simulink model "SwitchingDecisionMechanism_v02"  (R2021a)
settings: Solver=FixedStepAuto  StartTime=0.0  StopTime=inf  RelTol=1e-3
model workspace (MAT data in the model file):
  SL_ROS_VariableLengthArrays_MaxSizes.CommonInfo.ArrayTruncateAction = 'EmitWarning'
  SL_ROS_VariableLengthArrays_MaxSizes.MsgTypeMap = containers.Map
  SL_ROS_VariableLengthArrays_MaxSizes.MsgTypeMap.serialization.keys = {'sensor_msgs/LaserScan'}
  SL_ROS_VariableLengthArrays_MaxSizes.MsgTypeMap.serialization.values{1}(1).PropertyName = 'Intensities'
  SL_ROS_VariableLengthArrays_MaxSizes.MsgTypeMap.serialization.values{1}(1).DataType = 'single'
  SL_ROS_VariableLengthArrays_MaxSizes.MsgTypeMap.serialization.values{1}(1).MaxLength = 1084
  SL_ROS_VariableLengthArrays_MaxSizes.MsgTypeMap.serialization.values{1}(2).PropertyName = 'Ranges'
  SL_ROS_VariableLengthArrays_MaxSizes.MsgTypeMap.serialization.values{1}(2).DataType = 'single'
  SL_ROS_VariableLengthArrays_MaxSizes.MsgTypeMap.serialization.values{1}(2).MaxLength = 1084
  SL_ROS_VariableLengthArrays_MaxSizes.MsgTypeMap.serialization.uniformity = 0
  SL_ROS_VariableLengthArrays_MaxSizes.MsgTypeMap.serialization.keyType = 'char'
  SL_ROS_VariableLengthArrays_MaxSizes.MsgTypeMap.serialization.valueType = 'any'
libraries: robotlib x3
settings Model: Creator=roboticlab01  LastModifiedBy=roboticlab02
settings SolverCC: AlgebraicLoopSolver=TrustRegion
settings OptimizationCC: EnhancedBackFolding=on  PassReuseOutputArgsAs=Individual arguments  MaxStackSize=64  OptimizeBlockOrder=speed  DifferentSizesBufferReuse=on  OptimizationCustomize=off  EfficientTunableParamExpr=on
settings DebuggingCC: ParameterTunabilityLossMsg=error  SFMachineParentedDataDiag=warning
settings HardwareCC: ProdBitPerPointer=32  ProdBitPerSizeT=32  ProdBitPerPtrDiffT=32  ProdLargestAtomicFloat=None  ProdIntDivRoundTo=Undefined  ProdEndianess=Unspecified  ProdWordSize=32  ProdHWDeviceType=Generic->Unspecified (assume 32-bit Generic)
settings SFSimCC: MATLABDynamicMemAlloc=off  CustomCodeUndefinedFunction=UseInterfaceOnly  SimTargetLang=C++
settings RTWCC: SystemTargetFile=ert.tlc  HardwareBoard=Robot Operating System (ROS)  TLCOptions="-aInlineSetEventsForThisBaseRateFcn=TLC_FALSE -aSuppressMultiTaskScheduler=TLC_FALSE  -aRateBasedStepFcn=0"  TemplateMakefile=ert_default_tmf  GenerateReport=on  Toolchain=Catkin  IncludeHyperlinkInReport=on  LaunchReport=on  TargetLang=C++  GenerateTraceInfo=on  GenerateTraceReport=on  GenerateTraceReportSl=on  GenerateTraceReportSf=on  GenerateTraceReportEml=on
settings CodeAppCC: ForceParamTrailComments=on  IgnoreCustomStorageClasses=off  OperatorAnnotations=on  SimulinkDataObjDesc=on  SFDataObjDesc=on  InsertBlockDesc=on
settings ERTTargetCC: SupportVariableSizeSignals=on

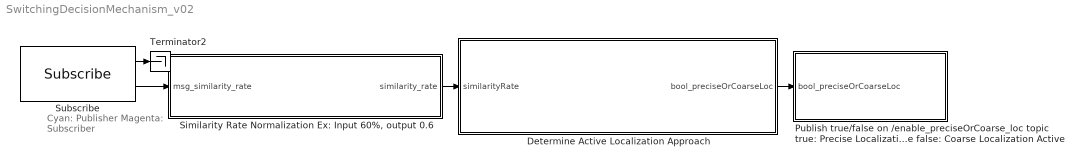
== system SwitchingDecisionMechanism_v02 ==
  note: Cyan: Publisher
      | Magenta: Subscriber
  Determine Active Localization Approach : Subsystem
  Publish true/false on /enable_preciseOrCoarse_loc topic true: Precise Localization Active false: Coarse Localization Active : Subsystem
  "Similarity Rate Normalization Ex: Input 60%, output 0.6" : Subsystem
  Subscribe : robotlib/Subscribe  topicSource=Specify your own  topic=/similarity_rate_corr  messageType=std_msgs/Int16  SampleTime=-1  legacyBusStruct=off  messageQueueLength=1
  Terminator2 : Terminator
  wires:
  Subscribe/1 -> Terminator2/1
  Subscribe/2 -> "Similarity Rate Normalization Ex: Input 60%, output 0.6"/1(msg_similarity_rate)
  "Similarity Rate Normalization Ex: Input 60%, output 0.6"/1(similarity_rate) -> Determine Active Localization Approach/1(similarityRate)
  Determine Active Localization Approach/1(bool_preciseOrCoarseLoc) -> Publish true/false on /enable_preciseOrCoarse_loc topic true: Precise Localization Active false: Coarse Localization Active/1(bool_preciseOrCoarseLoc)

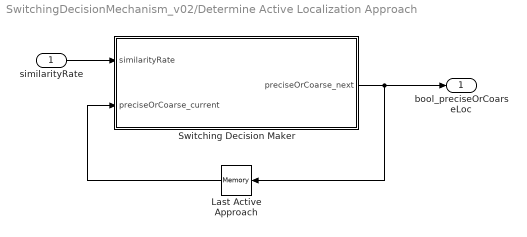
== system SwitchingDecisionMechanism_v02/Determine Active Localization Approach ==
  similarityRate : Inport
  Last Active Approach : Memory  InitialCondition=false(1)
  Switching Decision Maker : MATLAB Function  TreatAsAtomicUnit=on
  bool_preciseOrCoarseLoc : Outport
  wires:
  Switching Decision Maker/1(preciseOrCoarse_next) -> bool_preciseOrCoarseLoc/1, Last Active Approach/1
  similarityRate/1 -> Switching Decision Maker/1(similarityRate)
  Last Active Approach/1 -> Switching Decision Maker/2(preciseOrCoarse_current)

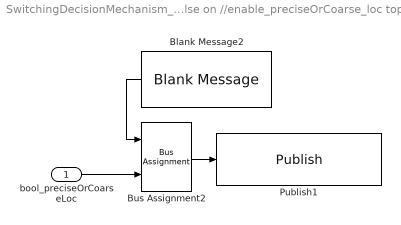
== system SwitchingDecisionMechanism_v02/Publish true//false on //enable_preciseOrCoarse_loc topic true: Precise Localization Active false: Coarse Localization Active ==
  bool_preciseOrCoarseLoc : Inport
  Blank Message2 : robotlib/Blank Message  messageClass=Message  entityType=std_msgs/Bool  messageType=std_msgs/Bool  SampleTime=inf  legacyBusStruct=off
      settings: SourceProductBaseCode=RO
  Bus Assignment2 : BusAssignment  AssignedSignals=Data
  Publish1 : robotlib/Publish  topicSource=Specify your own  topic=/enable_preciseOrCoarse_loc  messageType=std_msgs/Bool  legacyBusStruct=off  messageQueueLength=1
      settings: SourceProductBaseCode=RO
  wires:
  Bus Assignment2/1 -> Publish1/1
  bool_preciseOrCoarseLoc/1 -> Bus Assignment2/2
  Blank Message2/1 -> Bus Assignment2/1

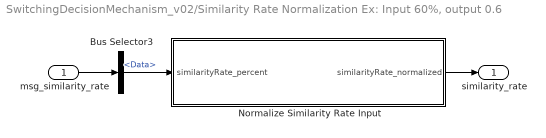
== system SwitchingDecisionMechanism_v02/Similarity Rate Normalization Ex: Input 60%, output 0.6 ==
  msg_similarity_rate : Inport
  Bus Selector3 : BusSelector  OutputSignals=Data
  Normalize Similarity Rate Input : MATLAB Function  TreatAsAtomicUnit=on
  similarity_rate : Outport
  wires:
  Bus Selector3/1 -> Normalize Similarity Rate Input/1(similarityRate_percent)  "<Data>"
  msg_similarity_rate/1 -> Bus Selector3/1
  Normalize Similarity Rate Input/1(similarityRate_normalized) -> similarity_rate/1

== matlab function SwitchingDecisionMechanism_v02/Determine Active Localization Approach/Switching Decision Maker ==
  data: similarityRate input; preciseOrCoarse_current input; preciseOrCoarse_next output
function preciseOrCoarse_next = SwitchOrNot(similarityRate,preciseOrCoarse_current)
    if preciseOrCoarse_current % if precise localization is active
        if similarityRate > 0.65
            preciseOrCoarse_next = true(1); % precise localization enabled
        else
            preciseOrCoarse_next = false(1); % coarse localization enabled
        end
    elseif ~preciseOrCoarse_current
        if similarityRate > 0.75
            preciseOrCoarse_next = true(1); % precise localization enabled
        else
            preciseOrCoarse_next = false(1); % coarse localization enabled
        end
    else
        preciseOrCoarse_next = false(1); % coarse localization enabled
    end
end

== matlab function SwitchingDecisionMechanism_v02/Similarity Rate Normalization Ex: Input 60%, output 0.6/Normalize Similarity Rate Input ==
  data: similarityRate_percent input; similarityRate_normalized output size=1 [..2000]
function similarityRate_normalized   = SimilarityRateNormalize(similarityRate_percent)
    if isempty(similarityRate_percent) || isnan(similarityRate_percent) || isinf(similarityRate_percent) || similarityRate_percent < 0 || similarityRate_percent > 100
        similarityRate_normalized = double(0.5); % default value 50 percent
    else
        similarityRate_normalized = double(similarityRate_percent)/100;
    end
end
